simulink model "Simulink"  (R2020b)
settings: Solver=FixedStepAuto  StartTime=0.0  StopTime=50  FixedStep=0.001  RelTol=1e-3
values from neighbouring files (symbols this model uses):
  A = [3 1 2;4 2 1;-2 -1 -1]    [main.m]
  A34_plus = A34'*inv(A34*A34')    [main.m]
  B = [0;2;1]    [main.m]
  G = blkdiag(T2,1)*T1    [main.m]
  K = y/X    [main.m]
  Kline = Anew(3,:)    [main.m]
  mui = 0.5    [main.m]
  P = inv(X)    [main.m]
  PHI = eye(3)    [main.m]
  x0 = [-1;5;3]    [main.m]
settings Model: Creator=sokra  LastModifiedBy=sokra

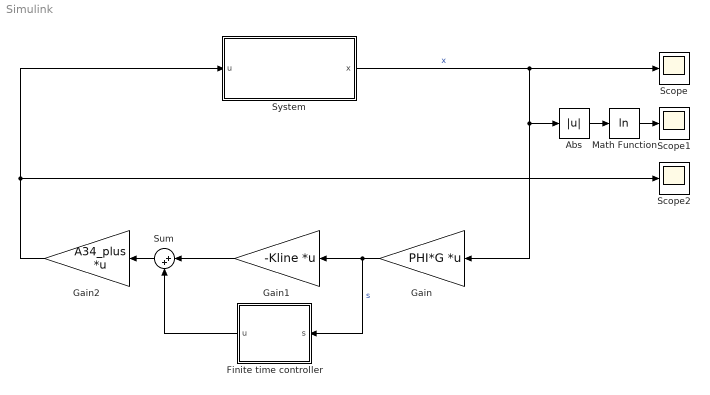
== system Simulink ==
  Abs : Abs
  Finite time controller : MATLAB Function  TreatAsAtomicUnit=on
  Gain : Gain  Gain=PHI*G  Multiplication=Matrix(K*u)
  Gain1 : Gain  Gain=-Kline  Multiplication=Matrix(K*u)
  Gain2 : Gain  Gain=A34_plus  Multiplication=Matrix(K*u)
  Math Function : Math  Operator=log  SaturateOnIntegerOverflow=on
  Scope : Scope
  Scope1 : Scope
  Scope2 : Scope
  Sum : Sum  Inputs=|++
  System : Subsystem
  wires:
  System/1(x) -> Abs/1, Gain/1, Scope/1  "x"
  Gain/1 -> Finite time controller/1(s), Gain1/1  "s"
  Gain2/1 -> System/1(u), Scope2/1
  Finite time controller/1(u) -> Sum/2
  Sum/1 -> Gain2/1
  Gain1/1 -> Sum/1
  Abs/1 -> Math Function/1
  Math Function/1 -> Scope1/1

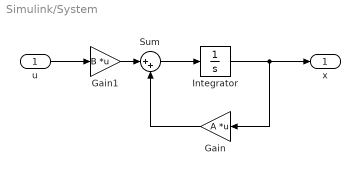
== system Simulink/System ==
  u : Inport
  Gain : Gain  Gain=A  Multiplication=Matrix(K*u)
  Gain1 : Gain  Gain=B  Multiplication=Matrix(K*u)
  Integrator : Integrator  InitialCondition=x0
  Sum : Sum  Inputs=|++
  x : Outport
  wires:
  Sum/1 -> Integrator/1
  Gain1/1 -> Sum/1
  Integrator/1 -> x/1, Gain/1
  Gain/1 -> Sum/2
  u/1 -> Gain1/1

== matlab function Simulink/Finite time controller ==
  data: u output size=1; s input; P parameter; mui parameter; K parameter
function u = fcn(s,P, mui,K)
%This function is used to create the finite time stibilization command
%P, mui,K,Vmax, Vmin are parameters definied at the main program
%s is the state variable for the system after applying the Block
%Decomposition method
% This function represents the implicity Lyaponuv function Q
f=@(x)(s'*[x^(-1-2*mui) 0 0;0 x^(-1-1*mui) 0;0 0 x^(-1)]*P*[x^(-1-2*mui) 0 0;0 x^(-1-1*mui) 0;0 0 x^(-1)]*s-1);
% Algorithm to find V correspond to input s
Vmin=0.000005;
a=0.001;
b=20;
for i=1:1:1000
if(f(b)>0)
    a=b;b=2*b;
elseif (f(a)<0)
    b=a;a=max(a/2,Vmin);
else
    c=(a+b)/2;
    if(f(c)<0)
        b=c;
    else
        a=max(c,Vmin);
    end
end
if (abs(b-a)<0.000001)
    break;
end
end
V=b;
%control signal
u=V^(1-mui)*K*[V^(-1-2*mui) 0 0;0 V^(-1-1*mui) 0;0 0 V^(-1)]*s;
